simulink model "E_Transmission_Loss_Through_channel"  (R2020a)
settings: Solver=VariableStepAuto  StartTime=0.0  StopTime=10.0  RelTol=1e-3
settings Model: Creator=Abdullah Abdelaziz  LastModifiedBy=Abdullah Abdelaziz

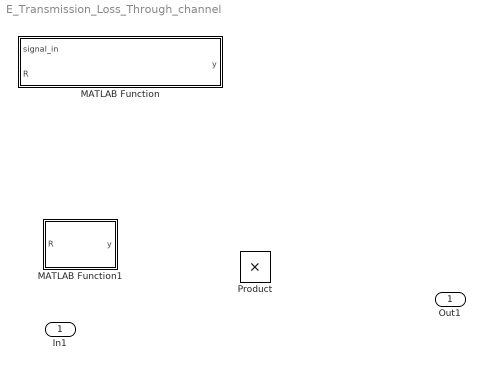
== system E_Transmission_Loss_Through_channel ==
  In1 : Inport
  MATLAB Function : MATLAB Function  TreatAsAtomicUnit=on
  MATLAB Function1 : MATLAB Function  TreatAsAtomicUnit=on
  Product : Product
  Out1 : Outport

== matlab function E_Transmission_Loss_Through_channel/MATLAB Function ==
  data: signal_in input; y output; R input
function y = attenuate_by_range(signal_in, R)
% This function correctly attenuates the signal amplitude based on 
% spherical spreading, where amplitude is proportional to 1/R.

% --- Input Arguments ---
% signal_in: The input signal from the transmitter
% R:         The range (distance) in meters

% --- Output Argument ---
% y:         The attenuated output signal

% Ensure R is not zero to prevent a "divide by zero" error.
% If R is 0, we use 'eps', which is the smallest possible number in MATLAB.
if R <= 0
    R = eps; 
end

% The attenuation factor is 1 divided by the range.
attenuation_factor = 1/R;

% Multiply the input signal by the attenuation factor.
y = signal_in * attenuation_factor;

end

== matlab function E_Transmission_Loss_Through_channel/MATLAB Function1 ==
  data: R input; y output
function y = attenuation_using_range(R)

loss_factor = 20 * log10(R);
y = loss_factor;

end
